simulink model "replayMPCData"  (R2018b)
settings: Solver=VariableStepAuto  StartTime=0.0  StopTime=inf  RelTol=1e-3
libraries: etargetslib x1, dspnetwork x1
settings Model: Creator=ge34qer  LastModifiedBy=ge34qer

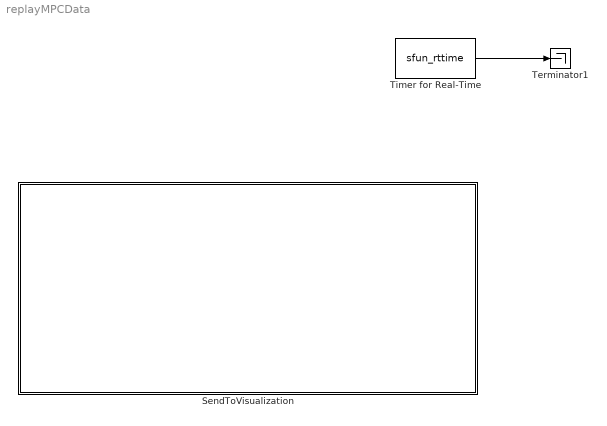
== system replayMPCData ==
  SendToVisualization : Subsystem
  Terminator1 : Terminator
  Timer for Real-Time : S-Function  FunctionName=sfun_rttime  Parameters=1  SFunctionDeploymentMode=off  EnableBusSupport=off
  wires:
  Timer for Real-Time/1 -> Terminator1/1

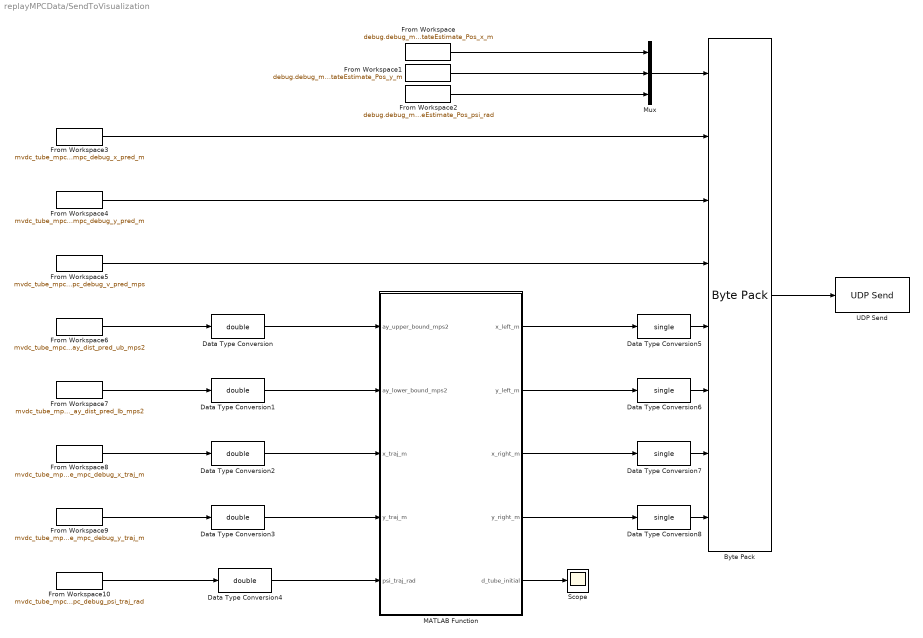
== system replayMPCData/SendToVisualization ==
  Byte Pack : etargetslib/Byte Pack  datatypes={'double', 'single', 'single', 'single', 'single', 'single', 'single', 'single'}  byteAlign=1
  Data Type Conversion{,1..4} (5 alike) : DataTypeConversion  OutDataTypeStr=double
  Data Type Conversion{5..8} (4 alike) : DataTypeConversion  OutDataTypeStr=single
  From Workspace : FromWorkspace  VariableName=debug.debug_mvdc_state_estimation_debug_StateEstimate_Pos_x_m  SampleTime=0
  From Workspace1 : FromWorkspace  VariableName=debug.debug_mvdc_state_estimation_debug_StateEstimate_Pos_y_m  SampleTime=0
  From Workspace10 : FromWorkspace  VariableName=mvdc_tube_mpc_debug.mvdc_tube_mpc_debug_psi_traj_rad  SampleTime=0
  From Workspace2 : FromWorkspace  VariableName=debug.debug_mvdc_state_estimation_debug_StateEstimate_Pos_psi_rad  SampleTime=0
  From Workspace3 : FromWorkspace  VariableName=mvdc_tube_mpc_debug.mvdc_tube_mpc_debug_x_pred_m  SampleTime=0
  From Workspace4 : FromWorkspace  VariableName=mvdc_tube_mpc_debug.mvdc_tube_mpc_debug_y_pred_m  SampleTime=0
  From Workspace5 : FromWorkspace  VariableName=mvdc_tube_mpc_debug.mvdc_tube_mpc_debug_v_pred_mps  SampleTime=0
  From Workspace6 : FromWorkspace  VariableName=mvdc_tube_mpc_debug.mvdc_tube_mpc_debug_ay_dist_pred_ub_mps2  SampleTime=0
  From Workspace7 : FromWorkspace  VariableName=mvdc_tube_mpc_debug.mvdc_tube_mpc_debug_ay_dist_pred_lb_mps2  SampleTime=0
  From Workspace8 : FromWorkspace  VariableName=mvdc_tube_mpc_debug.mvdc_tube_mpc_debug_x_traj_m  SampleTime=0
  From Workspace9 : FromWorkspace  VariableName=mvdc_tube_mpc_debug.mvdc_tube_mpc_debug_y_traj_m  SampleTime=0
  MATLAB Function : MATLAB Function  TreatAsAtomicUnit=on
  Mux : Mux  Inputs=3
  Scope : Scope
  UDP Send : dspnetwork/UDP Send  remoteURL='127.0.0.1'  remotePort=5000  localURL='0.0.0.0'  localPortSource=Automatically determine  localPort=-1  sampletime=-1  blockPlatform=[]  separateLengthPort=0
      settings: SourceProductName=DSP System Toolbox  SourceProductBaseCode=DS
  wires:
  From Workspace4/1 -> Byte Pack/3
  Byte Pack/1 -> UDP Send/1
  From Workspace3/1 -> Byte Pack/2
  Mux/1 -> Byte Pack/1
  From Workspace5/1 -> Byte Pack/4
  From Workspace6/1 -> Data Type Conversion/1
  From Workspace7/1 -> Data Type Conversion1/1
  MATLAB Function/1(x_left_m) -> Data Type Conversion5/1
  MATLAB Function/2(y_left_m) -> Data Type Conversion6/1
  MATLAB Function/3(x_right_m) -> Data Type Conversion7/1
  MATLAB Function/4(y_right_m) -> Data Type Conversion8/1
  Data Type Conversion/1 -> MATLAB Function/1(ay_upper_bound_mps2)
  Data Type Conversion1/1 -> MATLAB Function/2(ay_lower_bound_mps2)
  Data Type Conversion2/1 -> MATLAB Function/3(x_traj_m)
  Data Type Conversion3/1 -> MATLAB Function/4(y_traj_m)
  Data Type Conversion4/1 -> MATLAB Function/5(psi_traj_rad)
  Data Type Conversion5/1 -> Byte Pack/5
  Data Type Conversion6/1 -> Byte Pack/6
  Data Type Conversion7/1 -> Byte Pack/7
  Data Type Conversion8/1 -> Byte Pack/8
  From Workspace8/1 -> Data Type Conversion2/1
  From Workspace9/1 -> Data Type Conversion3/1
  From Workspace10/1 -> Data Type Conversion4/1
  MATLAB Function/5(d_tube_initial) -> Scope/1
  From Workspace/1 -> Mux/1
  From Workspace1/1 -> Mux/2
  From Workspace2/1 -> Mux/3

== matlab function replayMPCData/SendToVisualization/MATLAB Function ==
  data: ay_upper_bound_mps2 input; x_left_m output; ay_lower_bound_mps2 input; x_traj_m input; y_traj_m input; psi_traj_rad input; y_left_m output; x_right_m output; y_right_m output; d_tube_initial output
function [x_left_m, y_left_m, x_right_m, y_right_m, d_tube_initial] = fcn(ay_upper_bound_mps2, ay_lower_bound_mps2, x_traj_m, y_traj_m, psi_traj_rad)

% initialize outputs
x_left_m = zeros(50, 1); 
y_left_m = zeros(50, 1);
x_right_m = zeros(50, 1);
y_right_m = zeros(50, 1);

A_d = [1.0000,         0,         0;...
         0,    1.0000,    0.0400;
         0,         0,    1.0000]; 
B_d = [0.0400,         0;...
         0,         0;...
         0,    0.0400]; 
K_t = [-4.6094,    0, 0; ...
    0.0000,  -4,   -4]; 

dist_ay_spread = (ay_upper_bound_mps2(1) - ay_lower_bound_mps2(1))/2; 

% generate matrix for shape matrices to be stored in
Q_s = zeros(3,3*50);
d_tube_pred = zeros(50, 1); 

Q = @(Qs) (A_d + B_d*K_t)*Qs*(A_d+ B_d*K_t)';
Q_tilde = B_d*diag([1^2, dist_ay_spread^2])*B_d';    
% define minkowski sum
Q_sum = @(Q1,Q2) (1 + sqrt(trace(Q2)/max(1e-7,trace(Q1))))*Q1+...
          (1 + sqrt(trace(Q1)/max(1e-7,trace(Q2))))*Q2;
% get initial tube size
Qs = diag([0.05^2, 0.02^2, 0.05^2]);

% set initial tube size
Q_s(1:3,1:3) = Qs;
for i = 2:50
        Qs = Q_sum(Q(Qs), Q_tilde);
        Q_s(:,(i-1)*3+1:(i-1)*3+3) = Qs;            
end    

for j=1:1:50
    d_tube_pred(j) = sqrt([0 1 0]*Q_s(1:3,(j-1)*3+1:(j-1)*3+3)*[0;1;0]); 
end

% transform everything to cartesian coordinates
for j = 1:1:50
    x_left_m(j) = x_traj_m(j) - sin(psi_traj_rad(j) + pi/2)*d_tube_pred(j); 
    y_left_m(j) = y_traj_m(j) + cos(psi_traj_rad(j) + pi/2)*d_tube_pred(j); 
    x_right_m(j) = x_traj_m(j) + sin(psi_traj_rad(j) + pi/2)*d_tube_pred(j); 
    y_right_m(j) = y_traj_m(j) - cos(psi_traj_rad(j) + pi/2)*d_tube_pred(j); 
end

d_tube_initial = dist_ay_spread;
